simulink model "LgrstOpnLStEnCtrl"  (R2018b)
settings: Solver=FixedStepDiscrete  StartTime=0.0  StopTime=10.0  FixedStep=0.01  RelTol=1e-3
undefined symbols (not defined in the file or in its folder): data, KeSMSw4SSecRwLtStLgrstUpwdDnwdOpenPos1_Val, SecRwLtStFtrstEn_Clear, SecRwLtStFtrstEn_Set, SecRwLtStFwdBkwdEn_Clear, SecRwLtStFwdBkwdEn_Set, SecRwLtStLgrstInwdOtwdEn_Clear, SecRwLtStLgrstInwdOtwdEn_Set, SecRwLtStLgrstUpwdDnwdEn_Clear, SecRwLtStLgrstUpwdDnwdEn_Set
libraries: simulink x10
settings Model: ModifiedHistory="2023.11.16  V2.3.0 Issue 566045 全躺，vip，腿托打开增加前后位置"  Creator=sn2xws  LastModifiedBy=sn2xws
settings DataIOCC: SaveFormat=StructureWithTime
settings OptimizationCC: DefaultParameterBehavior=Inlined  EnhancedBackFolding=on  PassReuseOutputArgsAs=Individual arguments  ZeroExternalMemoryAtStartup=off  ZeroInternalMemoryAtStartup=off  OptimizeBlockOrder=speed  DifferentSizesBufferReuse=on  OptimizationCustomize=off
settings DebuggingCC: ParameterTunabilityLossMsg=error
settings ModelReferenceCC: ModelReferenceNumInstancesAllowed=Single
settings SFSimCC: MATLABDynamicMemAlloc=off
settings RTWCC: SystemTargetFile=autosar.tlc  GenCodeOnly=on  TemplateMakefile=ert_default_tmf  Description=AUTOSAR  GenerateReport=on  IncludeHyperlinkInReport=on  LaunchReport=on  GenerateTraceInfo=on  GenerateTraceReport=on  GenerateTraceReportSl=on  GenerateTraceReportSf=on  GenerateTraceReportEml=on  GenerateCodeMetricsReport=on
settings CodeAppCC: ForceParamTrailComments=on  IgnoreCustomStorageClasses=off  OperatorAnnotations=on  SimulinkDataObjDesc=on  SFDataObjDesc=on  InsertBlockDesc=on
settings STFCustomTargetCC: TargetLangStandard=C99 (ISO)  MultiwordLength=256  ParMdlRefBuildCompliant=on  CompOptLevelCompliant=on  IncludeMdlTerminateFcn=off  CombineOutputUpdateFcns=on  SuppressErrorStatus=on  ERTCustomFileBanners=on  SupportNonFinite=off  SupportComplex=off  SupportContinuousTime=off  SupportNonInlinedSFcns=off  RemoveResetFunc=on  MATLABClassNameForMDSCustomization=Simulink.SoftwareTarget.ERTCustomization  AutosarCompliant=on  UseToolchainInfoCompliant=on  LookupTableObjectStructAxisOrder=2,1,3,4,...  LUTObjectStructOrderEvenSpacing=Size,Table,Breakpoints  SystemTargetFile=autosar.tlc
settings ERTTargetCC: TargetLangStandard=C99 (ISO)  ConcurrentExecutionCompliant=off  IncludeMdlTerminateFcn=off  SuppressErrorStatus=on  SupportNonFinite=off  SupportComplex=off  ModelStepFunctionPrototypeControlCompliant=off  CPPClassGenCompliant=off  AutosarCompliant=on  LookupTableObjectStructAxisOrder=2,1,3,4,...  LUTObjectStructOrderEvenSpacing=Size,Table,Breakpoints  InlinedParameterPlacement=NonHierarchical  ERTCustomFileTemplate=example_file_process.tlc  ERTFilePackagingFormat=Compact

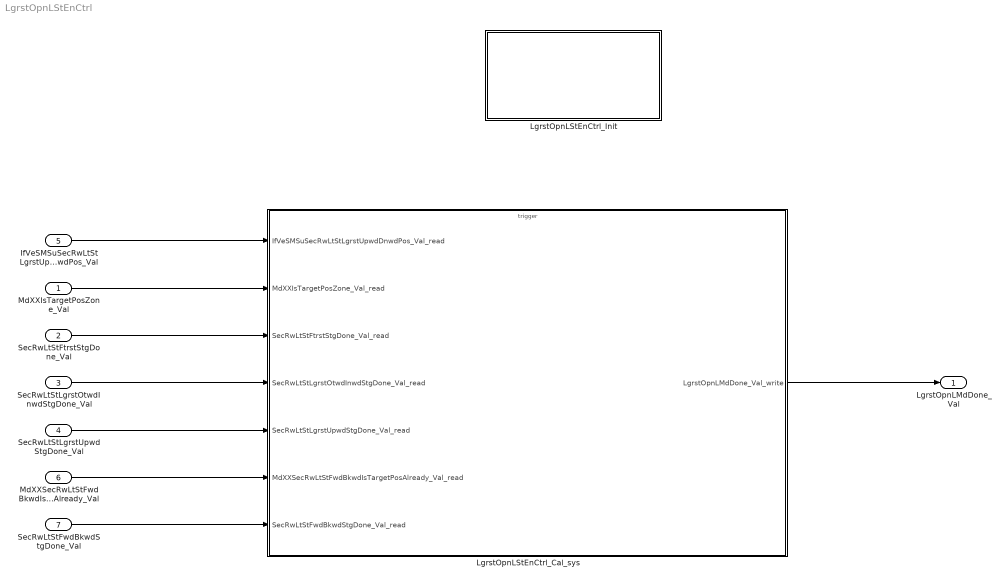
== system LgrstOpnLStEnCtrl ==
  MdXXIsTargetPosZone_Val : Inport  OutDataTypeStr=uint32  PortDimensions=1
  SecRwLtStFtrstStgDone_Val : Inport  Port=2  OutDataTypeStr=boolean  PortDimensions=1
  SecRwLtStLgrstOtwdInwdStgDone_Val : Inport  Port=3  OutDataTypeStr=boolean  PortDimensions=1
  SecRwLtStLgrstUpwdStgDone_Val : Inport  Port=4  OutDataTypeStr=boolean  PortDimensions=1
  IfVeSMSuSecRwLtStLgrstUpwdDnwdPos_Val : Inport  Port=5  OutDataTypeStr=uint16  PortDimensions=1
  MdXXSecRwLtStFwdBkwdIsTargetPosAlready_Val : Inport  Port=6  OutDataTypeStr=uint32  PortDimensions=1
  SecRwLtStFwdBkwdStgDone_Val : Inport  Port=7  OutDataTypeStr=boolean  PortDimensions=1
  LgrstOpnLStEnCtrl_Cal_sys : Subsystem
  LgrstOpnLStEnCtrl_Init : Subsystem
  LgrstOpnLMdDone_Val : Outport  OutDataTypeStr=uint8  PortDimensions=1
  wires:
  MdXXIsTargetPosZone_Val/1 -> LgrstOpnLStEnCtrl_Cal_sys/2(MdXXIsTargetPosZone_Val_read)
  SecRwLtStFtrstStgDone_Val/1 -> LgrstOpnLStEnCtrl_Cal_sys/3(SecRwLtStFtrstStgDone_Val_read)
  SecRwLtStLgrstOtwdInwdStgDone_Val/1 -> LgrstOpnLStEnCtrl_Cal_sys/4(SecRwLtStLgrstOtwdInwdStgDone_Val_read)
  SecRwLtStLgrstUpwdStgDone_Val/1 -> LgrstOpnLStEnCtrl_Cal_sys/5(SecRwLtStLgrstUpwdStgDone_Val_read)
  IfVeSMSuSecRwLtStLgrstUpwdDnwdPos_Val/1 -> LgrstOpnLStEnCtrl_Cal_sys/1(IfVeSMSuSecRwLtStLgrstUpwdDnwdPos_Val_read)
  LgrstOpnLStEnCtrl_Cal_sys/1(LgrstOpnLMdDone_Val_write) -> LgrstOpnLMdDone_Val/1
  MdXXSecRwLtStFwdBkwdIsTargetPosAlready_Val/1 -> LgrstOpnLStEnCtrl_Cal_sys/6(MdXXSecRwLtStFwdBkwdIsTargetPosAlready_Val_read)
  SecRwLtStFwdBkwdStgDone_Val/1 -> LgrstOpnLStEnCtrl_Cal_sys/7(SecRwLtStFwdBkwdStgDone_Val_read)

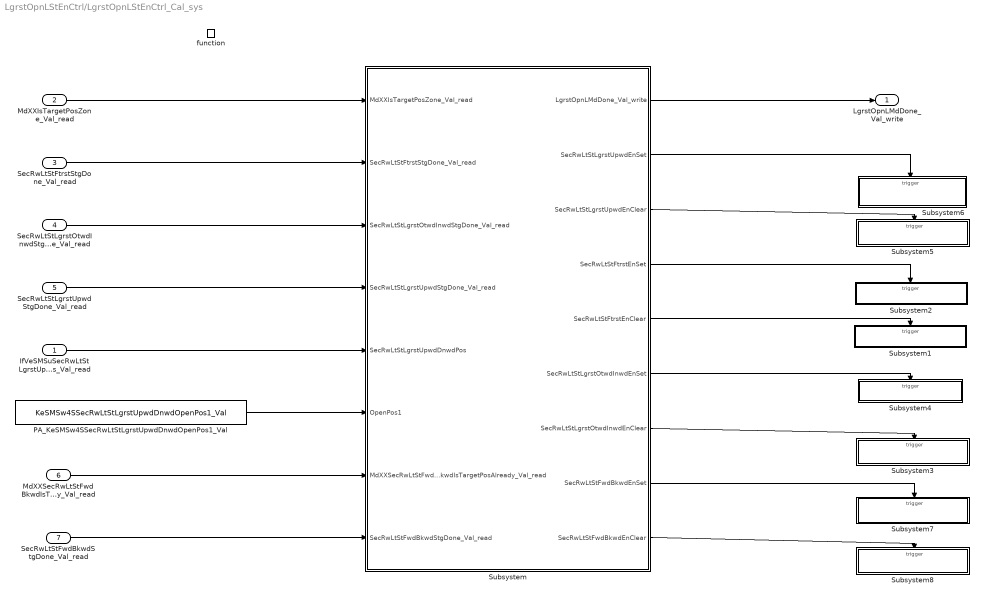
== system LgrstOpnLStEnCtrl/LgrstOpnLStEnCtrl_Cal_sys ==
  IfVeSMSuSecRwLtStLgrstUpwdDnwdPos_Val_read : Inport
  MdXXIsTargetPosZone_Val_read : Inport  Port=2
  SecRwLtStFtrstStgDone_Val_read : Inport  Port=3
  SecRwLtStLgrstOtwdInwdStgDone_Val_read : Inport  Port=4
  SecRwLtStLgrstUpwdStgDone_Val_read : Inport  Port=5
  MdXXSecRwLtStFwdBkwdIsTargetPosAlready_Val_read : Inport  Port=6
  SecRwLtStFwdBkwdStgDone_Val_read : Inport  Port=7
  function : TriggerPort  TriggerType=function-call  IsSimulinkFunction=on  FunctionName=LgrstOpnLStEnCtrl_Cal  VariantControl=(inherit)
  PA_KeSMSw4SSecRwLtStLgrstUpwdDnwdOpenPos1_Val : Constant  Value=KeSMSw4SSecRwLtStLgrstUpwdDnwdOpenPos1_Val
  Subsystem : Subsystem
  Subsystem1 : Subsystem
  Subsystem2 : Subsystem
  Subsystem3 : Subsystem
  Subsystem4 : Subsystem
  Subsystem5 : Subsystem
  Subsystem6 : Subsystem
  Subsystem7 : Subsystem
  Subsystem8 : Subsystem
  LgrstOpnLMdDone_Val_write : Outport
      settings: EnsureOutportIsVirtual=on
  wires:
  Subsystem/1(LgrstOpnLMdDone_Val_write) -> LgrstOpnLMdDone_Val_write/1
  Subsystem/6(SecRwLtStLgrstOtwdInwdEnSet) -> Subsystem4/Trigger
  Subsystem/3(SecRwLtStLgrstUpwdEnClear) -> Subsystem5/Trigger
  Subsystem/2(SecRwLtStLgrstUpwdEnSet) -> Subsystem6/Trigger
  Subsystem/7(SecRwLtStLgrstOtwdInwdEnClear) -> Subsystem3/Trigger
  Subsystem/5(SecRwLtStFtrstEnClear) -> Subsystem1/Trigger
  Subsystem/4(SecRwLtStFtrstEnSet) -> Subsystem2/Trigger
  PA_KeSMSw4SSecRwLtStLgrstUpwdDnwdOpenPos1_Val/1 -> Subsystem/6(OpenPos1)
  MdXXIsTargetPosZone_Val_read/1 -> Subsystem/1(MdXXIsTargetPosZone_Val_read)
  SecRwLtStFtrstStgDone_Val_read/1 -> Subsystem/2(SecRwLtStFtrstStgDone_Val_read)
  SecRwLtStLgrstOtwdInwdStgDone_Val_read/1 -> Subsystem/3(SecRwLtStLgrstOtwdInwdStgDone_Val_read)
  SecRwLtStLgrstUpwdStgDone_Val_read/1 -> Subsystem/4(SecRwLtStLgrstUpwdStgDone_Val_read)
  IfVeSMSuSecRwLtStLgrstUpwdDnwdPos_Val_read/1 -> Subsystem/5(SecRwLtStLgrstUpwdDnwdPos)
  MdXXSecRwLtStFwdBkwdIsTargetPosAlready_Val_read/1 -> Subsystem/7(MdXXSecRwLtStFwdBkwdIsTargetPosAlready_Val_read)
  SecRwLtStFwdBkwdStgDone_Val_read/1 -> Subsystem/8(SecRwLtStFwdBkwdStgDone_Val_read)
  Subsystem/8(SecRwLtStFwdBkwdEnSet) -> Subsystem7/Trigger
  Subsystem/9(SecRwLtStFwdBkwdEnClear) -> Subsystem8/Trigger

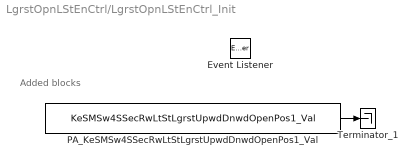
== system LgrstOpnLStEnCtrl/LgrstOpnLStEnCtrl_Init ==
  note: Added blocks
  Event Listener : EventListener  EventName=reset
  PA_KeSMSw4SSecRwLtStLgrstUpwdDnwdOpenPos1_Val : Constant  Value=KeSMSw4SSecRwLtStLgrstUpwdDnwdOpenPos1_Val
  Terminator_1 : Terminator
  wires:
  PA_KeSMSw4SSecRwLtStLgrstUpwdDnwdOpenPos1_Val/1 -> Terminator_1/1

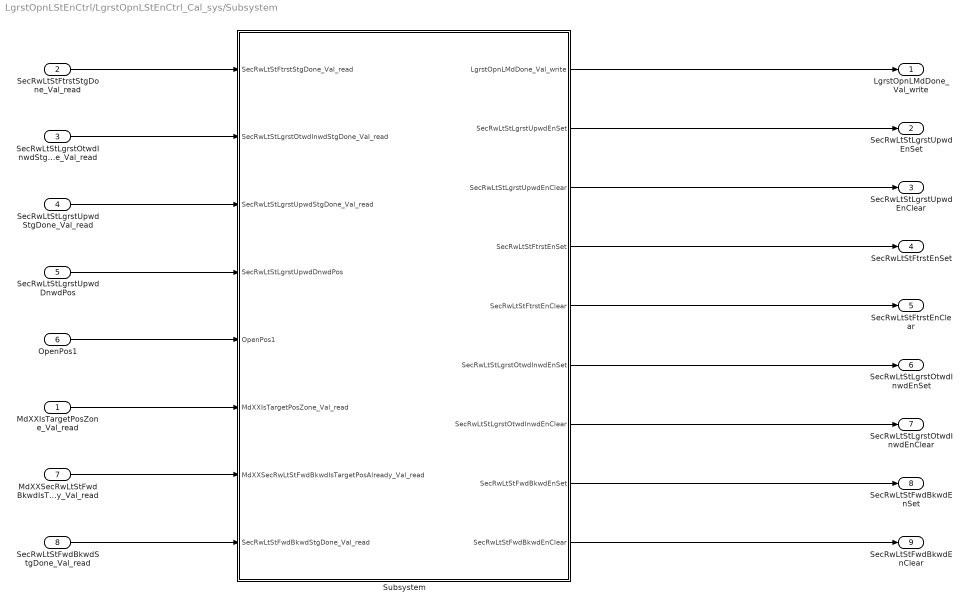
== system LgrstOpnLStEnCtrl/LgrstOpnLStEnCtrl_Cal_sys/Subsystem ==
  MdXXIsTargetPosZone_Val_read : Inport
  SecRwLtStFtrstStgDone_Val_read : Inport  Port=2
  SecRwLtStLgrstOtwdInwdStgDone_Val_read : Inport  Port=3
  SecRwLtStLgrstUpwdStgDone_Val_read : Inport  Port=4
  SecRwLtStLgrstUpwdDnwdPos : Inport  Port=5
  OpenPos1 : Inport  Port=6
  MdXXSecRwLtStFwdBkwdIsTargetPosAlready_Val_read : Inport  Port=7
  SecRwLtStFwdBkwdStgDone_Val_read : Inport  Port=8
  Subsystem : Subsystem
  LgrstOpnLMdDone_Val_write : Outport
      settings: EnsureOutportIsVirtual=on
  SecRwLtStLgrstUpwdEnSet : Outport  Port=2
  SecRwLtStLgrstUpwdEnClear : Outport  Port=3
  SecRwLtStFtrstEnSet : Outport  Port=4
  SecRwLtStFtrstEnClear : Outport  Port=5
  SecRwLtStLgrstOtwdInwdEnSet : Outport  Port=6
  SecRwLtStLgrstOtwdInwdEnClear : Outport  Port=7
  SecRwLtStFwdBkwdEnSet : Outport  Port=8
  SecRwLtStFwdBkwdEnClear : Outport  Port=9
  wires:
  SecRwLtStFtrstStgDone_Val_read/1 -> Subsystem/1(SecRwLtStFtrstStgDone_Val_read)
  SecRwLtStLgrstOtwdInwdStgDone_Val_read/1 -> Subsystem/2(SecRwLtStLgrstOtwdInwdStgDone_Val_read)
  SecRwLtStLgrstUpwdStgDone_Val_read/1 -> Subsystem/3(SecRwLtStLgrstUpwdStgDone_Val_read)
  Subsystem/1(LgrstOpnLMdDone_Val_write) -> LgrstOpnLMdDone_Val_write/1
  MdXXIsTargetPosZone_Val_read/1 -> Subsystem/6(MdXXIsTargetPosZone_Val_read)
  Subsystem/3(SecRwLtStLgrstUpwdEnClear) -> SecRwLtStLgrstUpwdEnClear/1
  Subsystem/4(SecRwLtStFtrstEnSet) -> SecRwLtStFtrstEnSet/1
  Subsystem/2(SecRwLtStLgrstUpwdEnSet) -> SecRwLtStLgrstUpwdEnSet/1
  Subsystem/5(SecRwLtStFtrstEnClear) -> SecRwLtStFtrstEnClear/1
  Subsystem/6(SecRwLtStLgrstOtwdInwdEnSet) -> SecRwLtStLgrstOtwdInwdEnSet/1
  Subsystem/7(SecRwLtStLgrstOtwdInwdEnClear) -> SecRwLtStLgrstOtwdInwdEnClear/1
  SecRwLtStLgrstUpwdDnwdPos/1 -> Subsystem/4(SecRwLtStLgrstUpwdDnwdPos)
  OpenPos1/1 -> Subsystem/5(OpenPos1)
  SecRwLtStFwdBkwdStgDone_Val_read/1 -> Subsystem/8(SecRwLtStFwdBkwdStgDone_Val_read)
  MdXXSecRwLtStFwdBkwdIsTargetPosAlready_Val_read/1 -> Subsystem/7(MdXXSecRwLtStFwdBkwdIsTargetPosAlready_Val_read)
  Subsystem/8(SecRwLtStFwdBkwdEnSet) -> SecRwLtStFwdBkwdEnSet/1
  Subsystem/9(SecRwLtStFwdBkwdEnClear) -> SecRwLtStFwdBkwdEnClear/1

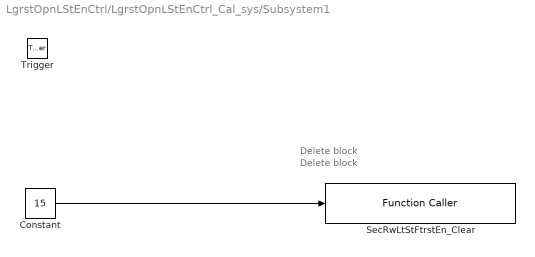
== system LgrstOpnLStEnCtrl/LgrstOpnLStEnCtrl_Cal_sys/Subsystem1 ==
  note: Delete block
  note: Delete block
  Trigger : TriggerPort  TriggerType=function-call  VariantControl=Variant  StatesWhenEnabling=reset  PortDimensions=1
  Constant : Constant  Value=15  OutDataTypeStr=uint8
  SecRwLtStFtrstEn_Clear : FunctionCaller  FunctionPrototype=SecRwLtStFtrstEn_Clear(data)  InputArgumentSpecifications=uint8(1)
  wires:
  Constant/1 -> SecRwLtStFtrstEn_Clear/1

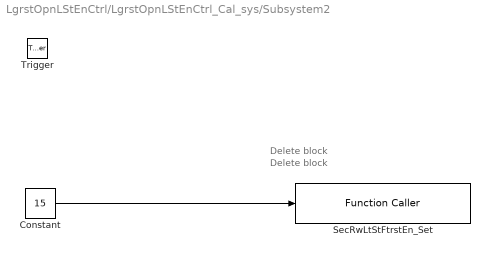
== system LgrstOpnLStEnCtrl/LgrstOpnLStEnCtrl_Cal_sys/Subsystem2 ==
  note: Delete block
  note: Delete block
  Trigger : TriggerPort  TriggerType=function-call  VariantControl=Variant  StatesWhenEnabling=reset  PortDimensions=1
  Constant : Constant  Value=15  OutDataTypeStr=uint8
  SecRwLtStFtrstEn_Set : FunctionCaller  FunctionPrototype=SecRwLtStFtrstEn_Set(data)  InputArgumentSpecifications=uint8(1)
  wires:
  Constant/1 -> SecRwLtStFtrstEn_Set/1

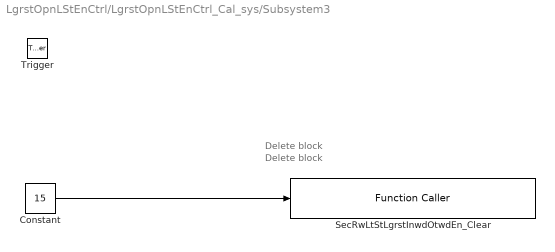
== system LgrstOpnLStEnCtrl/LgrstOpnLStEnCtrl_Cal_sys/Subsystem3 ==
  note: Delete block
  note: Delete block
  Trigger : TriggerPort  TriggerType=function-call  VariantControl=Variant  StatesWhenEnabling=reset  PortDimensions=1
  Constant : Constant  Value=15  OutDataTypeStr=uint8
  SecRwLtStLgrstInwdOtwdEn_Clear : FunctionCaller  FunctionPrototype=SecRwLtStLgrstInwdOtwdEn_Clear(data)  InputArgumentSpecifications=uint8(1)
  wires:
  Constant/1 -> SecRwLtStLgrstInwdOtwdEn_Clear/1

== system LgrstOpnLStEnCtrl/LgrstOpnLStEnCtrl_Cal_sys/Subsystem4 ==
  note: Delete block
  note: Delete block
  Trigger : TriggerPort  TriggerType=function-call  VariantControl=Variant  StatesWhenEnabling=reset  PortDimensions=1
  Constant : Constant  Value=15  OutDataTypeStr=uint8
  SecRwLtStLgrstInwdOtwdEn_Set : FunctionCaller  FunctionPrototype=SecRwLtStLgrstInwdOtwdEn_Set(data)  InputArgumentSpecifications=uint8(1)
  wires:
  Constant/1 -> SecRwLtStLgrstInwdOtwdEn_Set/1

== system LgrstOpnLStEnCtrl/LgrstOpnLStEnCtrl_Cal_sys/Subsystem5 ==
  note: Delete block
  note: Delete block
  Trigger : TriggerPort  TriggerType=function-call  VariantControl=Variant  StatesWhenEnabling=reset  PortDimensions=1
  Constant : Constant  Value=15  OutDataTypeStr=uint8
  SecRwLtStLgrstUpwdDnwdEn_Clear : FunctionCaller  FunctionPrototype=SecRwLtStLgrstUpwdDnwdEn_Clear(data)  InputArgumentSpecifications=uint8(1)
  wires:
  Constant/1 -> SecRwLtStLgrstUpwdDnwdEn_Clear/1

== system LgrstOpnLStEnCtrl/LgrstOpnLStEnCtrl_Cal_sys/Subsystem6 ==
  note: Delete block
  note: Delete block
  Trigger : TriggerPort  TriggerType=function-call  VariantControl=Variant  StatesWhenEnabling=reset  PortDimensions=1
  Constant : Constant  Value=15  OutDataTypeStr=uint8
  SecRwLtStLgrstUpwdDnwdEn_Set : FunctionCaller  FunctionPrototype=SecRwLtStLgrstUpwdDnwdEn_Set(data)  InputArgumentSpecifications=uint8(1)
  wires:
  Constant/1 -> SecRwLtStLgrstUpwdDnwdEn_Set/1

== system LgrstOpnLStEnCtrl/LgrstOpnLStEnCtrl_Cal_sys/Subsystem7 ==
  note: Delete block
  Trigger : TriggerPort  TriggerType=function-call  VariantControl=Variant  StatesWhenEnabling=reset  PortDimensions=1
  Constant : Constant  Value=15  OutDataTypeStr=uint8
  SecRwLtStFwdBkwdEn_Set : FunctionCaller  FunctionPrototype=SecRwLtStFwdBkwdEn_Set(data)  InputArgumentSpecifications=uint8(1)
  wires:
  Constant/1 -> SecRwLtStFwdBkwdEn_Set/1

== system LgrstOpnLStEnCtrl/LgrstOpnLStEnCtrl_Cal_sys/Subsystem8 ==
  note: Delete block
  Trigger : TriggerPort  TriggerType=function-call  VariantControl=Variant  StatesWhenEnabling=reset  PortDimensions=1
  Constant : Constant  Value=15  OutDataTypeStr=uint8
  SecRwLtStFwdBkwdEn_Clear : FunctionCaller  FunctionPrototype=SecRwLtStFwdBkwdEn_Clear(data)  InputArgumentSpecifications=uint8(1)
  wires:
  Constant/1 -> SecRwLtStFwdBkwdEn_Clear/1

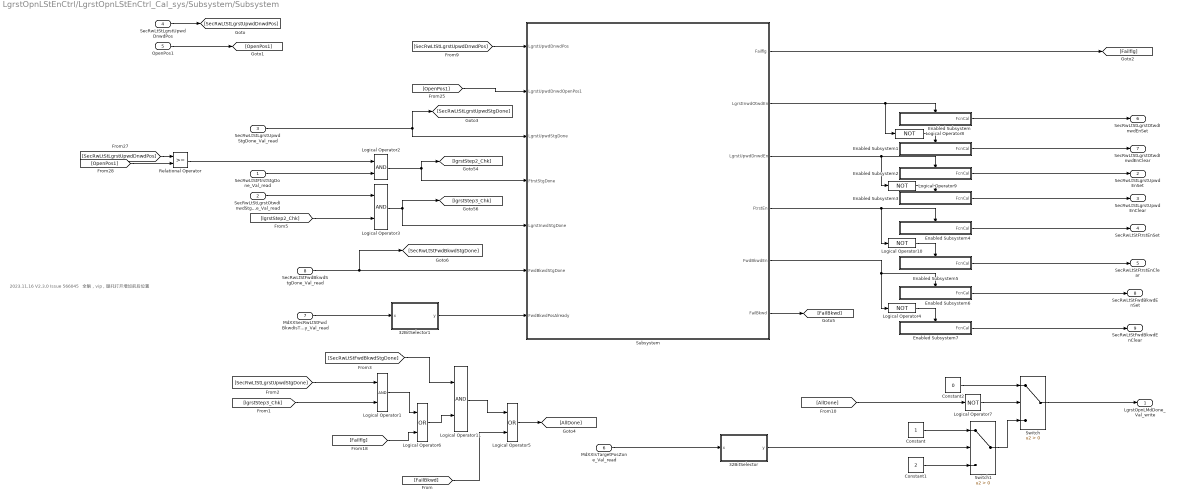
== system LgrstOpnLStEnCtrl/LgrstOpnLStEnCtrl_Cal_sys/Subsystem/Subsystem ==
  note: 2023.11.16 V2.3.0 Issue 566045 全躺，vip，腿托打开增加前后位置
  SecRwLtStFtrstStgDone_Val_read : Inport
  SecRwLtStLgrstOtwdInwdStgDone_Val_read : Inport  Port=2
  SecRwLtStLgrstUpwdStgDone_Val_read : Inport  Port=3
  SecRwLtStLgrstUpwdDnwdPos : Inport  Port=4
  OpenPos1 : Inport  Port=5
  MdXXIsTargetPosZone_Val_read : Inport  Port=6
  MdXXSecRwLtStFwdBkwdIsTargetPosAlready_Val_read : Inport  Port=7
  SecRwLtStFwdBkwdStgDone_Val_read : Inport  Port=8
  32BitSelector : Subsystem  mask(32 Bit Selector){BitNum=15}
      mask prompts: BitNum "Select Bit Number"
      mask help: Allows selection of a particular bit (0-31) out of a packed word up to 32 bits long. Output will be true if the bit number selected via the mask parameter is equal to one.
      mask TypeOptions BitNum: 0 | 1 | 2 | 3 | 4 | 5 | 6 | 7 | 8 | 9 | 10 | 11 | 12 | 13 | 14 | 15 | 16 | 17 | 18 | 19 | 20 | 21 | 22 | 23 | 24 | 25 | 26 | 27 | 28 | 29 | 30 | 31
      mask Display:
      | text(0.5, 0.8,'BIT','horizontalAlignment','center')
      | text(0.5, 0.5,'SELECTOR','horizontalAlignment','center')
      | text(0.5, 0.2,['-- Bit ',char(get_param(gcb,'BitNum')),' --'],'horizontalAlignment','center')
  32BitSelector1 : Subsystem  mask(32 Bit Selector){BitNum=15}
      mask prompts: BitNum "Select Bit Number"
      mask help: Allows selection of a particular bit (0-31) out of a packed word up to 32 bits long. Output will be true if the bit number selected via the mask parameter is equal to one.
      mask TypeOptions BitNum: 0 | 1 | 2 | 3 | 4 | 5 | 6 | 7 | 8 | 9 | 10 | 11 | 12 | 13 | 14 | 15 | 16 | 17 | 18 | 19 | 20 | 21 | 22 | 23 | 24 | 25 | 26 | 27 | 28 | 29 | 30 | 31
      mask Display:
      | text(0.5, 0.8,'BIT','horizontalAlignment','center')
      | text(0.5, 0.5,'SELECTOR','horizontalAlignment','center')
      | text(0.5, 0.2,['-- Bit ',char(get_param(gcb,'BitNum')),' --'],'horizontalAlignment','center')
  Constant : Constant  OutDataTypeStr=uint8
  Constant1 : Constant  Value=2  OutDataTypeStr=uint8
  Constant2 : Constant  Value=0  OutDataTypeStr=uint8
  Enabled Subsystem : Subsystem  TreatAsAtomicUnit=on
  Enabled Subsystem1 : Subsystem  TreatAsAtomicUnit=on
  Enabled Subsystem2 : Subsystem  TreatAsAtomicUnit=on
  Enabled Subsystem3 : Subsystem  TreatAsAtomicUnit=on
  Enabled Subsystem4 : Subsystem  TreatAsAtomicUnit=on
  Enabled Subsystem5 : Subsystem  TreatAsAtomicUnit=on
  Enabled Subsystem6 : Subsystem  TreatAsAtomicUnit=on
  Enabled Subsystem7 : Subsystem  TreatAsAtomicUnit=on
  Logical Operator{1..3,11} (4 alike) : Logic  AllPortsSameDT=off  OutDataTypeStr=boolean
  Logical Operator{4,7..10} (5 alike) : Logic  Operator=NOT  AllPortsSameDT=off  OutDataTypeStr=boolean
  Logical Operator5 : Logic  Operator=OR  AllPortsSameDT=off  OutDataTypeStr=boolean
  Logical Operator6 : Logic  Operator=OR  AllPortsSameDT=off  OutDataTypeStr=boolean
  Relational Operator : RelationalOperator  OutDataTypeStr=boolean  RndMeth=Simplest
  Subsystem : Subsystem
  Switch : Switch  Criteria=u2 > Threshold
  Switch1 : Switch  Criteria=u2 > Threshold
  LgrstOpnLMdDone_Val_write : Outport
      settings: EnsureOutportIsVirtual=on
  SecRwLtStLgrstUpwdEnSet : Outport  Port=2
  SecRwLtStLgrstUpwdEnClear : Outport  Port=3
  SecRwLtStFtrstEnSet : Outport  Port=4
  SecRwLtStFtrstEnClear : Outport  Port=5
  SecRwLtStLgrstOtwdInwdEnSet : Outport  Port=6
  SecRwLtStLgrstOtwdInwdEnClear : Outport  Port=7
  SecRwLtStFwdBkwdEnSet : Outport  Port=8
  SecRwLtStFwdBkwdEnClear : Outport  Port=9
  wires:
  [SecRwLtStLgrstUpwdDnwdPos] -> Relational Operator/1
  [lgrstStep2_Chk] -> Logical Operator3/2
  SecRwLtStFtrstStgDone_Val_read/1 -> Logical Operator2/2
  Logical Operator3/1 -> [lgrstStep3_Chk], Subsystem/5(LgrstInwdStgDone)
  Logical Operator2/1 -> Subsystem/4(FtrstStgDone), [lgrstStep2_Chk]
  [OpenPos1] -> Relational Operator/2
  SecRwLtStLgrstOtwdInwdStgDone_Val_read/1 -> Logical Operator3/1
  SecRwLtStLgrstUpwdStgDone_Val_read/1 -> [SecRwLtStLgrstUpwdStgDone], Subsystem/3(LgrstUpwdStgDone)
  Relational Operator/1 -> Logical Operator2/1
  SecRwLtStLgrstUpwdDnwdPos/1 -> [SecRwLtStLgrstUpwdDnwdPos]
  OpenPos1/1 -> [OpenPos1]
  Logical Operator1/1 -> Logical Operator6/1
  [lgrstStep3_Chk] -> Logical Operator1/2
  [SecRwLtStLgrstUpwdStgDone] -> Logical Operator1/1
  [Failflg] -> Logical Operator6/2
  Logical Operator5/1 -> [AllDone]
  MdXXIsTargetPosZone_Val_read/1 -> 32BitSelector/1(x)
  Switch1/1 -> Switch/3
  Switch/1 -> LgrstOpnLMdDone_Val_write/1
  Logical Operator10/1 -> Enabled Subsystem5/Enable
  Logical Operator8/1 -> Enabled Subsystem1/Enable
  Logical Operator9/1 -> Enabled Subsystem3/Enable
  Enabled Subsystem5/1(FcnCal) -> SecRwLtStFtrstEnClear/1
  Enabled Subsystem1/1(FcnCal) -> SecRwLtStLgrstOtwdInwdEnClear/1
  Enabled Subsystem2/1(FcnCal) -> SecRwLtStLgrstUpwdEnSet/1
  Enabled Subsystem4/1(FcnCal) -> SecRwLtStFtrstEnSet/1
  Enabled Subsystem/1(FcnCal) -> SecRwLtStLgrstOtwdInwdEnSet/1
  Enabled Subsystem3/1(FcnCal) -> SecRwLtStLgrstUpwdEnClear/1
  Logical Operator7/1 -> Switch/2
  [AllDone] -> Logical Operator7/1
  Constant2/1 -> Switch/1
  Constant1/1 -> Switch1/3
  Constant/1 -> Switch1/1
  32BitSelector/1(y) -> Switch1/2
  MdXXSecRwLtStFwdBkwdIsTargetPosAlready_Val_read/1 -> 32BitSelector1/1(x)
  Subsystem/2(LgrstInwdOtwdEn) -> Logical Operator8/1, Enabled Subsystem/Enable
  Subsystem/3(LgrstUpwdDnwdEn) -> Enabled Subsystem2/Enable, Logical Operator9/1
  Subsystem/4(FtrstEn) -> Enabled Subsystem4/Enable, Logical Operator10/1
  [SecRwLtStLgrstUpwdDnwdPos] -> Subsystem/1(LgrstUpwdDnwdPos)
  [OpenPos1] -> Subsystem/2(LgrstUpwdDnwdOpenPos1)
  Subsystem/1(Failflg) -> [Failflg]
  Subsystem/5(FwdBkwdEn) -> Logical Operator4/1, Enabled Subsystem6/Enable
  Enabled Subsystem6/1(FcnCal) -> SecRwLtStFwdBkwdEnSet/1
  Enabled Subsystem7/1(FcnCal) -> SecRwLtStFwdBkwdEnClear/1
  Logical Operator4/1 -> Enabled Subsystem7/Enable
  32BitSelector1/1(y) -> Subsystem/7(FwdBkwdPosAlready)
  Subsystem/6(FailBkwd) -> [FailBkwd]
  [FailBkwd] -> Logical Operator5/2
  Logical Operator6/1 -> Logical Operator11/2
  SecRwLtStFwdBkwdStgDone_Val_read/1 -> [SecRwLtStFwdBkwdStgDone], Subsystem/6(FwdBkwdStgDone)
  [SecRwLtStFwdBkwdStgDone] -> Logical Operator11/1
  Logical Operator11/1 -> Logical Operator5/1

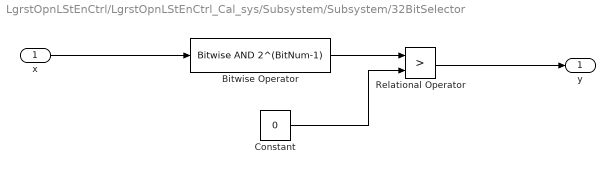
== system LgrstOpnLStEnCtrl/LgrstOpnLStEnCtrl_Cal_sys/Subsystem/Subsystem/32BitSelector ==
  x : Inport
  Bitwise Operator : simulink/Logic and Bit Operations/Bitwise Operator  logicop=AND  UseBitMask=on  BitMask=2^(BitNum-1)  BitMaskRealWorld=Stored Integer
  Constant : Constant  Value=0  OutDataTypeStr=uint32
  Relational Operator : RelationalOperator  Operator=>  OutDataTypeStr=boolean  RndMeth=Simplest
  y : Outport
  wires:
  Relational Operator/1 -> y/1
  Constant/1 -> Relational Operator/2
  x/1 -> Bitwise Operator/1
  Bitwise Operator/1 -> Relational Operator/1

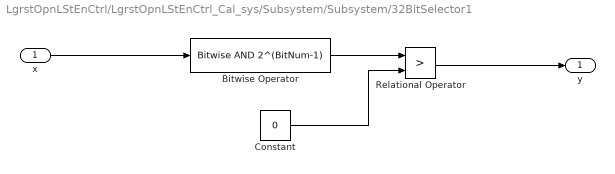
== system LgrstOpnLStEnCtrl/LgrstOpnLStEnCtrl_Cal_sys/Subsystem/Subsystem/32BitSelector1 ==
  x : Inport
  Bitwise Operator : simulink/Logic and Bit Operations/Bitwise Operator  logicop=AND  UseBitMask=on  BitMask=2^(BitNum-1)  BitMaskRealWorld=Stored Integer
  Constant : Constant  Value=0  OutDataTypeStr=uint32
  Relational Operator : RelationalOperator  Operator=>  OutDataTypeStr=boolean  RndMeth=Simplest
  y : Outport
  wires:
  Bitwise Operator/1 -> Relational Operator/1
  x/1 -> Bitwise Operator/1
  Constant/1 -> Relational Operator/2
  Relational Operator/1 -> y/1

== system LgrstOpnLStEnCtrl/LgrstOpnLStEnCtrl_Cal_sys/Subsystem/Subsystem/Enabled Subsystem ==
  Enable : EnablePort
  Function-Call Generator : simulink/Ports & Subsystems/Function-Call Generator  sample_time=-1  numberOfIterations=1
  FcnCal : Outport
  wires:
  Function-Call Generator/1 -> FcnCal/1

== system LgrstOpnLStEnCtrl/LgrstOpnLStEnCtrl_Cal_sys/Subsystem/Subsystem/Enabled Subsystem1 ==
  Enable : EnablePort
  Function-Call Generator : simulink/Ports & Subsystems/Function-Call Generator  sample_time=-1  numberOfIterations=1
  FcnCal : Outport
  wires:
  Function-Call Generator/1 -> FcnCal/1

== system LgrstOpnLStEnCtrl/LgrstOpnLStEnCtrl_Cal_sys/Subsystem/Subsystem/Enabled Subsystem2 ==
  Enable : EnablePort
  Function-Call Generator : simulink/Ports & Subsystems/Function-Call Generator  sample_time=-1  numberOfIterations=1
  FcnCal : Outport
  wires:
  Function-Call Generator/1 -> FcnCal/1

== system LgrstOpnLStEnCtrl/LgrstOpnLStEnCtrl_Cal_sys/Subsystem/Subsystem/Enabled Subsystem3 ==
  Enable : EnablePort
  Function-Call Generator : simulink/Ports & Subsystems/Function-Call Generator  sample_time=-1  numberOfIterations=1
  FcnCal : Outport
  wires:
  Function-Call Generator/1 -> FcnCal/1

== system LgrstOpnLStEnCtrl/LgrstOpnLStEnCtrl_Cal_sys/Subsystem/Subsystem/Enabled Subsystem4 ==
  Enable : EnablePort
  Function-Call Generator : simulink/Ports & Subsystems/Function-Call Generator  sample_time=-1  numberOfIterations=1
  FcnCal : Outport
  wires:
  Function-Call Generator/1 -> FcnCal/1

== system LgrstOpnLStEnCtrl/LgrstOpnLStEnCtrl_Cal_sys/Subsystem/Subsystem/Enabled Subsystem5 ==
  Enable : EnablePort
  Function-Call Generator : simulink/Ports & Subsystems/Function-Call Generator  sample_time=-1  numberOfIterations=1
  FcnCal : Outport
  wires:
  Function-Call Generator/1 -> FcnCal/1

== system LgrstOpnLStEnCtrl/LgrstOpnLStEnCtrl_Cal_sys/Subsystem/Subsystem/Enabled Subsystem6 ==
  Enable : EnablePort
  Function-Call Generator : simulink/Ports & Subsystems/Function-Call Generator  sample_time=-1  numberOfIterations=1
  FcnCal : Outport
  wires:
  Function-Call Generator/1 -> FcnCal/1

== system LgrstOpnLStEnCtrl/LgrstOpnLStEnCtrl_Cal_sys/Subsystem/Subsystem/Enabled Subsystem7 ==
  Enable : EnablePort
  Function-Call Generator : simulink/Ports & Subsystems/Function-Call Generator  sample_time=-1  numberOfIterations=1
  FcnCal : Outport
  wires:
  Function-Call Generator/1 -> FcnCal/1

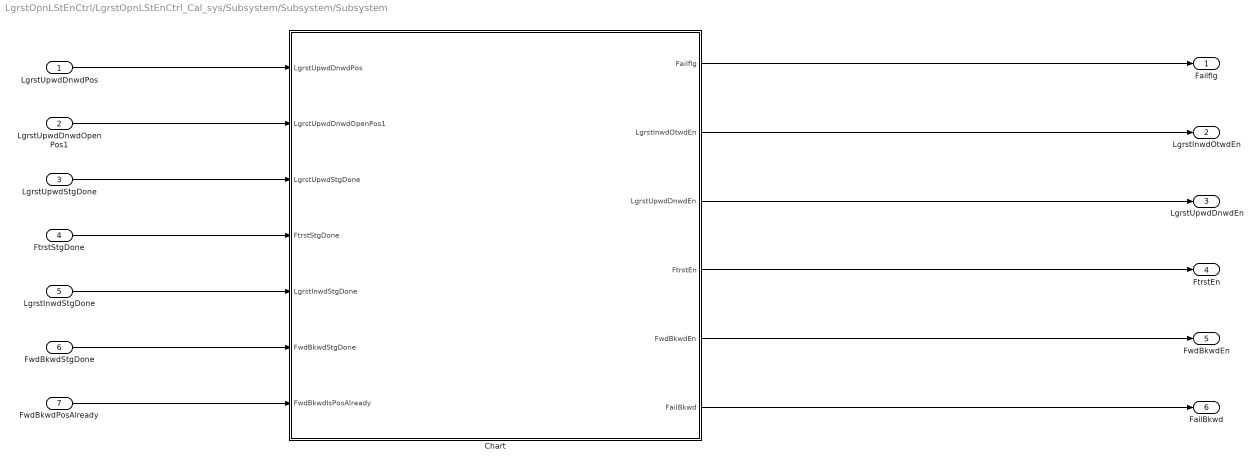
== system LgrstOpnLStEnCtrl/LgrstOpnLStEnCtrl_Cal_sys/Subsystem/Subsystem/Subsystem ==
  LgrstUpwdDnwdPos : Inport
  LgrstUpwdDnwdOpenPos1 : Inport  Port=2
  LgrstUpwdStgDone : Inport  Port=3
  FtrstStgDone : Inport  Port=4
  LgrstInwdStgDone : Inport  Port=5
  FwdBkwdStgDone : Inport  Port=6
  FwdBkwdPosAlready : Inport  Port=7
  Chart : Stateflow chart  TreatAsAtomicUnit=on
  Failflg : Outport
  LgrstInwdOtwdEn : Outport  Port=2
  LgrstUpwdDnwdEn : Outport  Port=3
  FtrstEn : Outport  Port=4
  FwdBkwdEn : Outport  Port=5
  FailBkwd : Outport  Port=6
  wires:
  LgrstUpwdDnwdPos/1 -> Chart/1(LgrstUpwdDnwdPos)
  LgrstUpwdDnwdOpenPos1/1 -> Chart/2(LgrstUpwdDnwdOpenPos1)
  LgrstUpwdStgDone/1 -> Chart/3(LgrstUpwdStgDone)
  LgrstInwdStgDone/1 -> Chart/5(LgrstInwdStgDone)
  FtrstStgDone/1 -> Chart/4(FtrstStgDone)
  Chart/1(Failflg) -> Failflg/1
  Chart/2(LgrstInwdOtwdEn) -> LgrstInwdOtwdEn/1
  Chart/3(LgrstUpwdDnwdEn) -> LgrstUpwdDnwdEn/1
  Chart/4(FtrstEn) -> FtrstEn/1
  Chart/5(FwdBkwdEn) -> FwdBkwdEn/1
  FwdBkwdStgDone/1 -> Chart/6(FwdBkwdStgDone)
  FwdBkwdPosAlready/1 -> Chart/7(FwdBkwdIsPosAlready)
  Chart/6(FailBkwd) -> FailBkwd/1

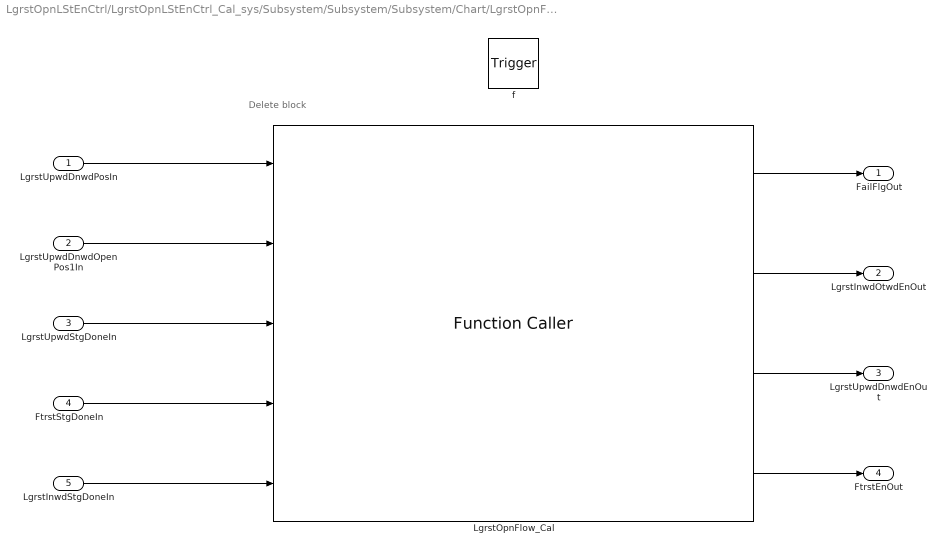
== system LgrstOpnLStEnCtrl/LgrstOpnLStEnCtrl_Cal_sys/Subsystem/Subsystem/Subsystem/Chart/LgrstOpnFlow_Cal ==
  note: Delete block
  LgrstUpwdDnwdPosIn : Inport
  LgrstUpwdDnwdOpenPos1In : Inport  Port=2
  LgrstUpwdStgDoneIn : Inport  Port=3
  FtrstStgDoneIn : Inport  Port=4
  LgrstInwdStgDoneIn : Inport  Port=5
  f : TriggerPort  TriggerType=function-call  VariantControl=(inherit)
      settings: CopyFcn=Stateflow.SLINSF.SimulinkMan.removeBlockPreDeleteFcn  PreDeleteFcn=Stateflow.SLINSF.SimulinkMan.unsafePredeleteFcn
  LgrstOpnFlow_Cal : FunctionCaller  FunctionPrototype=[Failflg,LgrstInwdOtwdEn,LgrstUpwdDnwdEn,FtrstEn] = LgrstOpnFlow_Cal(LgrstUpwdDnwdPos,LgrstUpwdDnwdOpenPos1,LgrstUpwdStgDone,FtrstStgDone,LgrstInwdStgDone)  InputArgumentSpecifications=uint16(1), uint16(1), boolean(true), boolean(true), boolean(true)  OutputArgumentSpecifications=boolean(true), boolean(true), boolean(true), boolean(true)
  FailFlgOut : Outport
  LgrstInwdOtwdEnOut : Outport  Port=2
  LgrstUpwdDnwdEnOut : Outport  Port=3
  FtrstEnOut : Outport  Port=4
  wires:
  LgrstUpwdDnwdPosIn/1 -> LgrstOpnFlow_Cal/1
  LgrstUpwdDnwdOpenPos1In/1 -> LgrstOpnFlow_Cal/2
  LgrstUpwdStgDoneIn/1 -> LgrstOpnFlow_Cal/3
  FtrstStgDoneIn/1 -> LgrstOpnFlow_Cal/4
  LgrstInwdStgDoneIn/1 -> LgrstOpnFlow_Cal/5
  LgrstOpnFlow_Cal/1 -> FailFlgOut/1
  LgrstOpnFlow_Cal/2 -> LgrstInwdOtwdEnOut/1
  LgrstOpnFlow_Cal/3 -> LgrstUpwdDnwdEnOut/1
  LgrstOpnFlow_Cal/4 -> FtrstEnOut/1

== stateflow chart LgrstOpnLStEnCtrl/LgrstOpnLStEnCtrl_Cal_sys/Subsystem/Subsystem/Subsystem/Chart ==
  state [FailFlgOut,LgrstInwdOtwdEnOut,LgrstUpwdDnwdEnOut,FtrstEnOut] = LgrstOpnFlow_Cal(LgrstUpwdDnwdPosIn,LgrstUpwdDnwdOpenPos1In,LgrstUpwdStgDoneIn,FtrstStgDoneIn,LgrstInwdStgDoneIn) [function]
  (default) -> (junction 11) : {
      | Failflg=0;
      | LgrstInwdOtwdEn=0;
      | LgrstUpwdDnwdEn=0;
      | FtrstEn=0;
      | FailBkwd=0;
      | }
  (junction 11) -> (junction 15) [order 1] : [!FwdBkwdStgDone]
  (junction 11) -> (junction 13) [order 2]
  (junction 15) -> (junction 42) : {FwdBkwdEn=1;}
  (junction 13) -> (junction 32) [order 1] : [!FwdBkwdIsPosAlready]
  (junction 13) -> (junction 39) [order 2] : {[Failflg,LgrstInwdOtwdEn,LgrstUpwdDnwdEn,FtrstEn] = LgrstOpnFlow_Cal(LgrstUpwdDnwdPos,LgrstUpwdDnwdOpenPos1,LgrstUpwdStgDone,FtrstStgDone,LgrstInwdStgDone);}
  (junction 32) -> (junction 41) : {FailBkwd=1;}
  (junction 41) -> (junction 42)
  (junction 42) -> (junction 34)
  (junction 34) -> (junction 39)
  (junction 39) -> (junction 45)
  data: FailFlgOut function_output; LgrstUpwdDnwdPosIn function_input; LgrstUpwdDnwdOpenPos1In function_input; LgrstUpwdStgDoneIn function_input; FtrstStgDoneIn function_input; LgrstInwdStgDoneIn function_input; LgrstInwdOtwdEnOut function_output; LgrstUpwdDnwdEnOut function_output; FtrstEnOut function_output; LgrstUpwdDnwdPos input; LgrstUpwdDnwdOpenPos1 input; LgrstUpwdStgDone input; FtrstStgDone input; LgrstInwdStgDone input; FwdBkwdStgDone input; FwdBkwdIsPosAlready input; Failflg output boolean; LgrstInwdOtwdEn output boolean; LgrstUpwdDnwdEn output boolean; FtrstEn output boolean; FwdBkwdEn output boolean; FailBkwd output boolean
